simulink model "Exp_07_03_01"  (R2012b)
settings: Solver=ode23tb  StartTime=0.0  StopTime=10.0  RelTol=1e-4
libraries: powerlib x8
settings Model: Creator=Abraham Xiao  LastModifiedBy=Abraham Xiao
settings RTWCC: GenerateReport=on  LaunchReport=on
settings CodeAppCC: ForceParamTrailComments=on  MATLABSourceComments=on

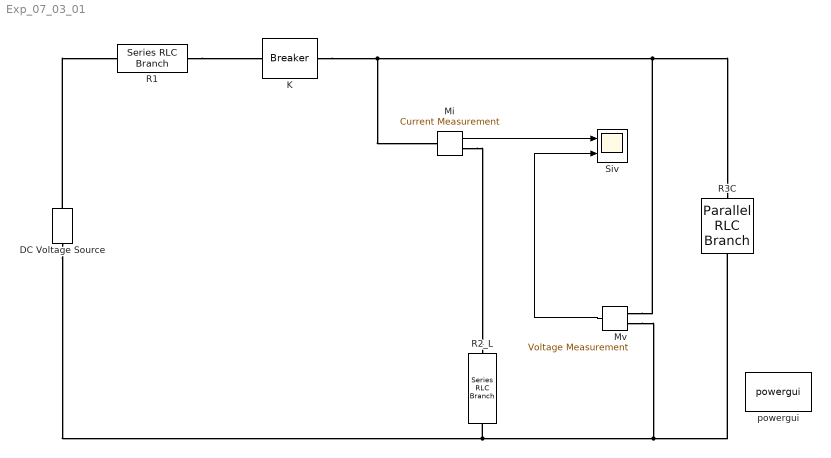
== system Exp_07_03_01 ==
  DC Voltage Source : powerlib/Electrical Sources/DC Voltage Source  Amplitude=10  Measurements=None
  K : powerlib/Elements/Breaker  BreakerResistance=0.01  InitialState=0  SnubberResistance=1e6  SnubberCapacitance=inf  SwitchingTimes=0  External=off  Measurements=None  MoreParameters=off  NoBreakLoop=off
  Mi : powerlib/Measurements/Current Measurement  PhasorSimulation=off  OutputType=Complex  PSBequivalent=0
  Mv : powerlib/Measurements/Voltage Measurement  PhasorSimulation=off  OutputType=Complex  PSBequivalent=0
  R1 : powerlib/Elements/Series RLC Branch  LConnTagsString=__new0  RConnTagsString=__new0  BranchType=R  Resistance=2  Inductance=1e-3  SetiL0=off  InitialCurrent=0  Capacitance=1e-6  Setx0=off  InitialVoltage=0  Measurements=None
  R2_L : powerlib/Elements/Series RLC Branch  LConnTagsString=__new0  RConnTagsString=__new0  BranchType=RL  Resistance=0.01  Inductance=0.3  SetiL0=on  InitialCurrent=1  Capacitance=1e-6  Setx0=off  InitialVoltage=0  Measurements=None
  R3C : powerlib/Elements/Parallel RLC Branch  LConnTagsString=a  RConnTagsString=__new0  BranchType=RC  Resistance=5  Inductance=1e-3  SetiL0=off  InitialCurrent=0  Capacitance=0.3  Setx0=on  InitialVoltage=-1  Measurements=None
  "Siv " : Scope  NumInputPorts=2
      settings: YMin=0~-2  YMax=7~3
  powergui : powerlib/powergui  Priority=1  SimulationMode=Continuous  SolverType=Tustin  SampleTime=50e-6  frequency=60  SPID=on  DisableSnubberDevices=on  DisableRonSwitches=on  DisableVfSwitches=off  SwTol=0  Interpol=off  DisplayEquations=on  FunctionMessages=off  frequencyindice=0  Pbase=100e6  ErrMax=1e-4  Iterations=50  UnitsV=kV  UnitsW=MW  echomessages=off  HookPort=off  EnableUseOfTLC=off  x0status=blocks  RestoreLinks=warning  ResistiveCurrentMeasurement=off  Ylog=off  Xlog=on  ShowGrid=off  save=off  variable=ZData  ZoomFFT=off  StartTime=0.0  cycles=1  DisplayStyle=1  FreqAxis=off  MaxFrequency=1000  frequencyindicesteady=1  display=off  methode=off
  wires:
  Mi/1 -> "Siv "/1
  Mv/1 -> "Siv "/2
  connections:
  DC Voltage Source/RConn1 -- R1/LConn1
  R1/RConn1 -- K/LConn1
  K/RConn1 -- Mv/LConn1 -- R3C/LConn1 -- Mi/LConn1
  Mi/RConn1 -- R2_L/LConn1
  DC Voltage Source/LConn1 -- Mv/LConn2 -- R3C/RConn1 -- R2_L/RConn1
